simulink model "PMLSM_CDL_MFAC_FFDLc"  (R2023a)
settings: Solver=VariableStepAuto  StartTime=0.0  StopTime=1  RelTol=1e-3
libraries: spsIGBTDiodeLib x6, spsVoltageMeasurementLib x3, slpidlib x2, spsDCVoltageSourceLib x1, simulink x1, spspowerguiLib x1
settings Model: SimulationMode=accelerator  Creator=ComeCross  LastModifiedBy=Administrator
settings SolverCC: ZeroCrossAlgorithm=Adaptive
settings DataIOCC: Refine=10
settings OptimizationCC: ReuseModelBlockBuffer=off
settings DebuggingCC: IgnoredZcDiagnostic=none

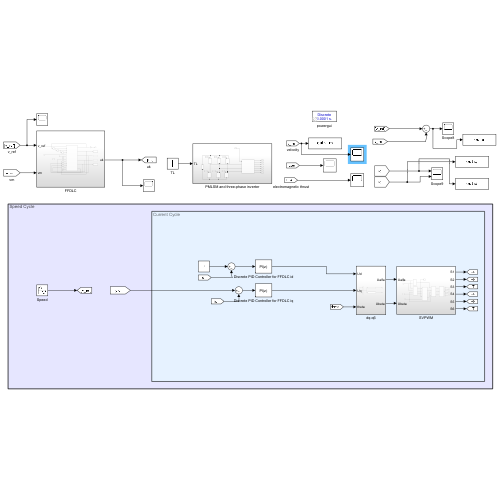
[thumbnail: Simulink's stored preview of the top-level diagram]
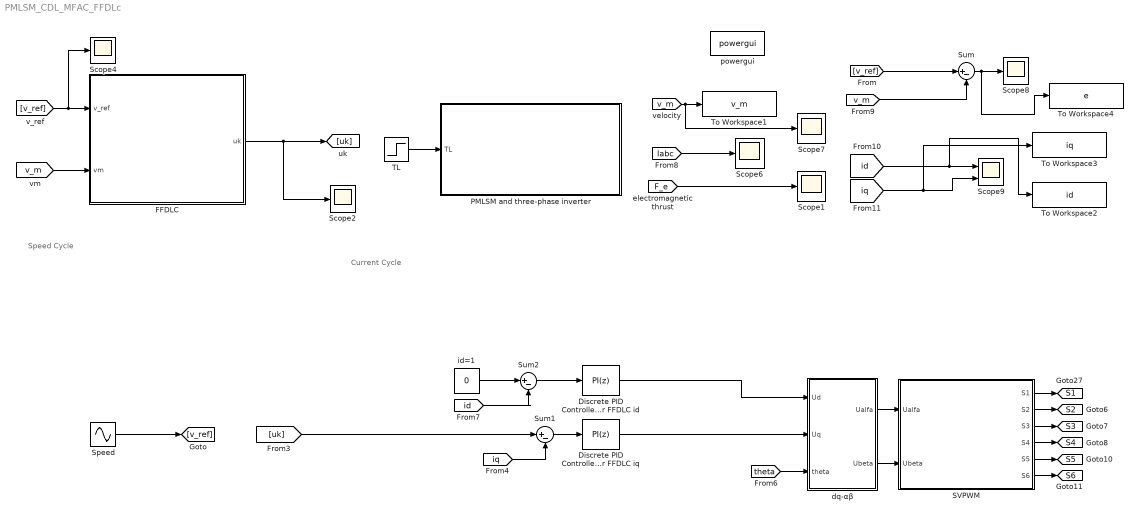
== system PMLSM_CDL_MFAC_FFDLc ==
  note: Speed Cycle
  note: Current Cycle
  Discrete PID Controller for FFDLC id : slpidlib/PID Controller  Controller=PI  Form=Parallel  TimeDomain=Discrete-time  UseExternalTs=off  SampleTime=1e-4  IntegratorMethod=Forward Euler  FilterMethod=Forward Euler  ControllerParametersSource=internal  P=1400  I=2400  UseKiTs=off  D=30  N=100  UseFilter=on  TunerSelectOption=Frequency Response Based  InitialConditionSource=internal  InitialConditionForIntegrator=0  InitialConditionForFilter=0  DifferentiatorICPrevScaledInput=0  ExternalReset=none  TrackingMode=off  Kt=1  LimitOutput=off  SatLimitsSource=internal  UpperSaturationLimit=inf  LowerSaturationLimit=-inf  LinearizeAsGain=off  AntiWindupMode=none  Kb=1  LimitIntegrator=off  UpperIntegratorSaturationLimit=inf  LowerIntegratorSaturationLimit=-inf  POutMin=[]  POutMax=[]  IOutMin=[]  IOutMax=[]  DOutMin=[]  DOutMax=[]  NOutMin=[]  NOutMax=[]  SumOutMin=[]  SumOutMax=[]  SaturationOutMin=[]  SaturationOutMax=[]  PParamMin=[]  PParamMax=[]  IParamMin=[]  IParamMax=[]  DParamMin=[]  DParamMax=[]  NParamMin=[]  NParamMax=[]  KbParamMin=[]  KbParamMax=[]  KtParamMin=[]  KtParamMax=[]  KbOutMin=[]  KbOutMax=[]  KtOutMin=[]  KtOutMax=[]  IntegratorOutMin=[]  IntegratorOutMax=[]  FilterOutMin=[]  FilterOutMax=[]  SumI1OutMin=[]  SumI1OutMax=[]  SumI2OutMin=[]  SumI2OutMax=[]  SumI3OutMin=[]  SumI3OutMax=[]  SumI4OutMin=[]  SumI4OutMax=[]  SumDOutMin=[]  SumDOutMax=[]  DifferentiatorOutMin=[]  DifferentiatorOutMax=[]  FilterDiffOutCoefMin=[]  FilterDiffOutCoefMax=[]  ReciprocalOutMin=[]  ReciprocalOutMax=[]  SumDenOutMin=[]  SumDenOutMax=[]  SumNumOutMin=[]  SumNumOutMax=[]  DivideOutMin=[]  DivideOutMax=[]  UdiffTsProdOutMin=[]  UdiffTsProdOutMax=[]  NTsProdOutMin=[]  NTsProdOutMax=[]  UintegralTsProdOutMin=[]  UintegralTsProdOutMax=[]  UngainTsProdOutMin=[]  UngainTsProdOutMax=[]  ClampingZeroOutDataTypeStr=Inherit: Inherit via back propagation  ClampingZeroOutMin=[]  ClampingZeroOutMax=[]  FilterDenConstantOutDataTypeStr=Inherit: Inherit via back propagation  FilterDenConstantOutMin=[]  FilterDenConstantOutMax=[]  PCopyOutDataTypeStr=Inherit: Inherit via back propagation  PCopyOutMin=[]  PCopyOutMax=[]  NCopyOutDataTypeStr=Inherit: Inherit via back propagation  NCopyOutMin=[]  NCopyOutMax=[]  IntegratorContinuousStateAttributes=''  IntegratorStateMustResolveToSignalObject=off  IntegratorRTWStateStorageClass=Auto  FilterContinuousStateAttributes=''  FilterStateMustResolveToSignalObject=off  FilterRTWStateStorageClass=Auto  ParallelPVariant=InternalParameters  IdealPVariant=Disabled  IVariant=InternalParameters  DVariant=Disabled  IntegratorVariant=Discrete  SatVariant=Disabled  AWVariant=Passthrough  PCopyVariant=Disabled  TRVariant=Disabled  FdbkBlocksVariant=Forward  IdealPFdbkVariant=Disabled  SatFdbkVariant=Disabled  DerivativeFilterVariant=Disabled  NVariant=Disabled  NCopyVariant=Disabled_SignalSpec  FilterICVariant=Disabled  IntegratorICVariant=InternalICs  ExternalResetVariant=Disabled  TRSumVariant=Passthrough  SumFdbkVariant=Disabled  SumVariant=Sum_PI  TsampFilterVariant=InternalTs  TsampNgainVariant=Passthrough  TsampIntegralVariant=Disabled_SignalSpec  ExternalSaturationOutDataTypeStr=Inherit: Same as second input
      settings: LibrarySourceBlock=simulink/Discrete/Discrete PID Controller
  Discrete PID Controller for FFDLC iq : slpidlib/PID Controller  Controller=PI  Form=Parallel  TimeDomain=Discrete-time  UseExternalTs=off  SampleTime=1e-4  IntegratorMethod=Forward Euler  FilterMethod=Forward Euler  ControllerParametersSource=internal  P=1400  I=2400  UseKiTs=off  D=30  N=100  UseFilter=on  TunerSelectOption=Frequency Response Based  InitialConditionSource=internal  InitialConditionForIntegrator=0  InitialConditionForFilter=0  DifferentiatorICPrevScaledInput=0  ExternalReset=none  TrackingMode=off  Kt=1  LimitOutput=off  SatLimitsSource=internal  UpperSaturationLimit=inf  LowerSaturationLimit=-inf  LinearizeAsGain=off  AntiWindupMode=none  Kb=1  LimitIntegrator=off  UpperIntegratorSaturationLimit=inf  LowerIntegratorSaturationLimit=-inf  POutMin=[]  POutMax=[]  IOutMin=[]  IOutMax=[]  DOutMin=[]  DOutMax=[]  NOutMin=[]  NOutMax=[]  SumOutMin=[]  SumOutMax=[]  SaturationOutMin=[]  SaturationOutMax=[]  PParamMin=[]  PParamMax=[]  IParamMin=[]  IParamMax=[]  DParamMin=[]  DParamMax=[]  NParamMin=[]  NParamMax=[]  KbParamMin=[]  KbParamMax=[]  KtParamMin=[]  KtParamMax=[]  KbOutMin=[]  KbOutMax=[]  KtOutMin=[]  KtOutMax=[]  IntegratorOutMin=[]  IntegratorOutMax=[]  FilterOutMin=[]  FilterOutMax=[]  SumI1OutMin=[]  SumI1OutMax=[]  SumI2OutMin=[]  SumI2OutMax=[]  SumI3OutMin=[]  SumI3OutMax=[]  SumI4OutMin=[]  SumI4OutMax=[]  SumDOutMin=[]  SumDOutMax=[]  DifferentiatorOutMin=[]  DifferentiatorOutMax=[]  FilterDiffOutCoefMin=[]  FilterDiffOutCoefMax=[]  ReciprocalOutMin=[]  ReciprocalOutMax=[]  SumDenOutMin=[]  SumDenOutMax=[]  SumNumOutMin=[]  SumNumOutMax=[]  DivideOutMin=[]  DivideOutMax=[]  UdiffTsProdOutMin=[]  UdiffTsProdOutMax=[]  NTsProdOutMin=[]  NTsProdOutMax=[]  UintegralTsProdOutMin=[]  UintegralTsProdOutMax=[]  UngainTsProdOutMin=[]  UngainTsProdOutMax=[]  ClampingZeroOutDataTypeStr=Inherit: Inherit via back propagation  ClampingZeroOutMin=[]  ClampingZeroOutMax=[]  FilterDenConstantOutDataTypeStr=Inherit: Inherit via back propagation  FilterDenConstantOutMin=[]  FilterDenConstantOutMax=[]  PCopyOutDataTypeStr=Inherit: Inherit via back propagation  PCopyOutMin=[]  PCopyOutMax=[]  NCopyOutDataTypeStr=Inherit: Inherit via back propagation  NCopyOutMin=[]  NCopyOutMax=[]  IntegratorContinuousStateAttributes=''  IntegratorStateMustResolveToSignalObject=off  IntegratorRTWStateStorageClass=Auto  FilterContinuousStateAttributes=''  FilterStateMustResolveToSignalObject=off  FilterRTWStateStorageClass=Auto  ParallelPVariant=InternalParameters  IdealPVariant=Disabled  IVariant=InternalParameters  DVariant=Disabled  IntegratorVariant=Discrete  SatVariant=Disabled  AWVariant=Passthrough  PCopyVariant=Disabled  TRVariant=Disabled  FdbkBlocksVariant=Forward  IdealPFdbkVariant=Disabled  SatFdbkVariant=Disabled  DerivativeFilterVariant=Disabled  NVariant=Disabled  NCopyVariant=Disabled_SignalSpec  FilterICVariant=Disabled  IntegratorICVariant=InternalICs  ExternalResetVariant=Disabled  TRSumVariant=Passthrough  SumFdbkVariant=Disabled  SumVariant=Sum_PI  TsampFilterVariant=InternalTs  TsampNgainVariant=Passthrough  TsampIntegralVariant=Disabled_SignalSpec  ExternalSaturationOutDataTypeStr=Inherit: Same as second input
      settings: LibrarySourceBlock=simulink/Discrete/Discrete PID Controller
  FFDLC : Subsystem
  PMLSM and three-phase inverter : Subsystem
  SVPWM : Subsystem
  Scope{1..2,4,6..8} (6 alike) : Scope
  Scope9 : Scope  NumInputPorts=2
  Speed : Sin  Amplitude=2  Frequency=10  SampleTime=0
  Sum : Sum  Inputs=|+-
  Sum1 : Sum  Inputs=|+-
  Sum2 : Sum  Inputs=|+-
  TL : Step  Time=0.2  SampleTime=1e-4
  To Workspace1 : ToWorkspace  VariableName=v_m  SaveFormat=Timeseries  SampleTime=-1
  To Workspace2 : ToWorkspace  VariableName=id  SaveFormat=Structure With Time  SampleTime=-1
  To Workspace3 : ToWorkspace  VariableName=iq  SaveFormat=Structure With Time  SampleTime=-1
  To Workspace4 : ToWorkspace  VariableName=e  SaveFormat=Structure With Time  SampleTime=-1
  dq-αβ : Subsystem
  id=1 : Constant  Value=0
  powergui : spspowerguiLib/powergui  Priority=1  SimulationMode=Discrete  SampleTime=1e-4  frequency=60  Iterations=50  frequencyindice=0  Pbase=100e6  ErrMax=1e-4  UnitsV=kV  UnitsW=MW  buscounter=0  FunctionMessages=off  echomessages=off  EnableUseOfTLC=off  CurrentSourceSwitches=off  DisableSnubberDevices=off  DisableRonSwitches=off  DisableVfSwitches=off  DisplayEquations=off  AutomaticDiscreteSolvers=off  SolverType=Tustin  Interpol=off  ExternalGateDelay=off  methode=off  Ts=0  x0status=blocks  SPID=off  SwTol=0  HookPort=off  NonlinearTolerance=1e-4  nMaxIteration=100  ContinueOnMaxIteration=off  RestoreLinks=warning  ResistiveCurrentMeasurement=off  Frange=[0:2:500]  Ylog=off  Xlog=on  ShowGrid=off  save=off  variable=ZData  structure=0  ZoomFFT=off  StartTime=0.0  cycles=1  DisplayStyle=1  fundamental=60  FreqAxis=off  MaxFrequency=1000  frequencyindicesteady=1  RmsSteady=1  display=off
  tag scope: S1=global, S2=global, S3=global, S4=global, S5=global, S6=global
  wires:
  [v_m] -> Scope7/1, To Workspace1/1
  [Iabc] -> Scope6/1
  [F_e] -> Scope1/1
  SVPWM/6(S6) -> [S6]
  [theta] -> dq-αβ/3(theta)
  SVPWM/5(S5) -> [S5]
  SVPWM/3(S3) -> [S3]
  SVPWM/1(S1) -> [S1]
  dq-αβ/2(Ubeta) -> SVPWM/2(Ubeta)
  SVPWM/4(S4) -> [S4]
  dq-αβ/1(Ualfa) -> SVPWM/1(Ualfa)
  SVPWM/2(S2) -> [S2]
  TL/1 -> PMLSM and three-phase inverter/1(TL)
  Speed/1 -> [v_ref]
  [v_ref] -> Scope4/1, FFDLC/1(v_ref)
  [v_m] -> FFDLC/2(vm)
  FFDLC/1(uk) -> [uk], Scope2/1
  [iq] -> Sum1/2
  Discrete PID Controller for FFDLC id/1 -> dq-αβ/1(Ud)
  id=1/1 -> Sum2/1
  [id] -> Sum2/2
  [v_ref] -> Sum/1
  [v_m] -> Sum/2
  Sum/1 -> To Workspace4/1, Scope8/1
  [id] -> To Workspace2/1, Scope9/1
  [iq] -> To Workspace3/1, Scope9/2
  Sum1/1 -> Discrete PID Controller for FFDLC iq/1
  Sum2/1 -> Discrete PID Controller for FFDLC id/1
  [uk] -> Sum1/1
  Discrete PID Controller for FFDLC iq/1 -> dq-αβ/2(Uq)

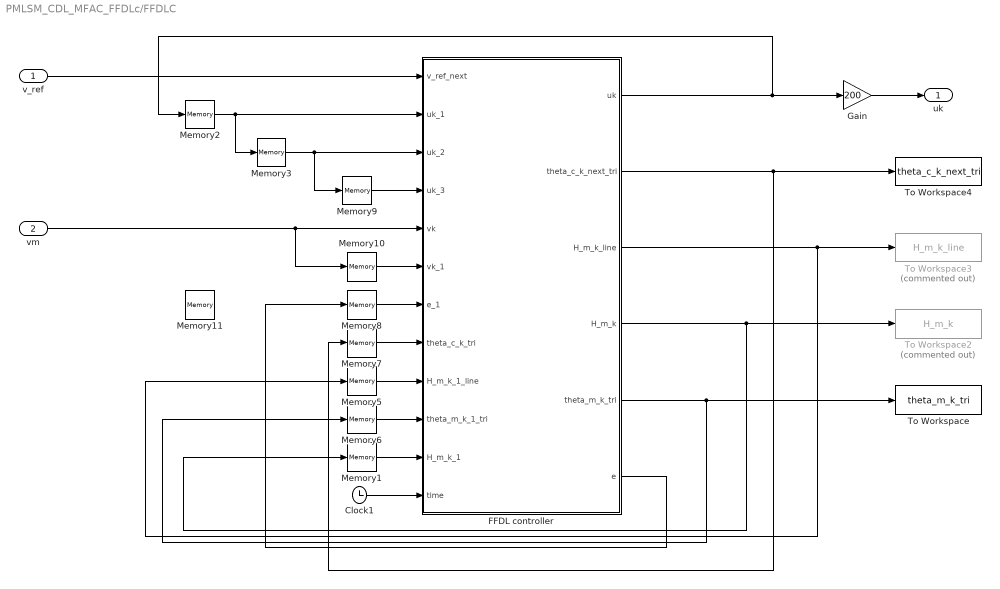
== system PMLSM_CDL_MFAC_FFDLc/FFDLC ==
  v_ref : Inport
  vm : Inport  Port=2
  Clock1 : Clock
  FFDL controller : MATLAB Function  TreatAsAtomicUnit=on
  Gain : Gain  Gain=200
  Memory1 : Memory  InitialCondition=[0.001,0.001,0]'  InheritSampleTime=on
  Memory10 : Memory  InitialCondition=[0]  InheritSampleTime=on
  Memory11 : Memory  InitialCondition=[0.0000]  InheritSampleTime=on
  Memory2 : Memory  InitialCondition=[0.0001]  InheritSampleTime=on
  Memory3 : Memory  InitialCondition=[0.0000]  InheritSampleTime=on
  Memory5 : Memory  InitialCondition=[0.0001,0.000]'  InheritSampleTime=on
  Memory6 : Memory  InitialCondition=[0.006,0.000,-0.000]'  InheritSampleTime=on  LinearizeAsDelay=on
  Memory7 : Memory  InitialCondition=[-0.0048,0.0001,0]'  InheritSampleTime=on
  Memory8 : Memory  InitialCondition=[0.000]  InheritSampleTime=on
  Memory9 : Memory  InitialCondition=[0.00]  InheritSampleTime=on
  To Workspace : ToWorkspace  VariableName=theta_m_k_tri  SaveFormat=Structure With Time  SampleTime=1e-4
      settings: MaxDataPoints=150000
  To Workspace2 : ToWorkspace  Commented=on  VariableName=H_m_k  SaveFormat=Structure With Time  SampleTime=1e-4
  To Workspace3 : ToWorkspace  Commented=on  VariableName=H_m_k_line  SaveFormat=Structure With Time  SampleTime=1e-4
  To Workspace4 : ToWorkspace  VariableName=theta_c_k_next_tri  SaveFormat=Structure With Time  SampleTime=1e-4
      settings: MaxDataPoints=150000
  uk : Outport
  wires:
  FFDL controller/2(theta_c_k_next_tri) -> Memory7/1, To Workspace4/1
  Memory3/1 -> Memory9/1, FFDL controller/3(uk_2)
  vm/1 -> Memory10/1, FFDL controller/5(vk)
  FFDL controller/1(uk) -> Memory2/1, Gain/1
  Memory2/1 -> FFDL controller/2(uk_1), Memory3/1
  FFDL controller/3(H_m_k_line) -> Memory5/1, To Workspace3/1
  FFDL controller/4(H_m_k) -> Memory1/1, To Workspace2/1
  FFDL controller/5(theta_m_k_tri) -> Memory6/1, To Workspace/1
  Memory9/1 -> FFDL controller/4(uk_3)
  v_ref/1 -> FFDL controller/1(v_ref_next)
  Memory10/1 -> FFDL controller/6(vk_1)
  FFDL controller/6(e) -> Memory8/1
  Memory8/1 -> FFDL controller/7(e_1)
  Memory7/1 -> FFDL controller/8(theta_c_k_tri)
  Memory5/1 -> FFDL controller/9(H_m_k_1_line)
  Memory6/1 -> FFDL controller/10(theta_m_k_1_tri)
  Memory1/1 -> FFDL controller/11(H_m_k_1)
  Gain/1 -> uk/1
  Clock1/1 -> FFDL controller/12(time)

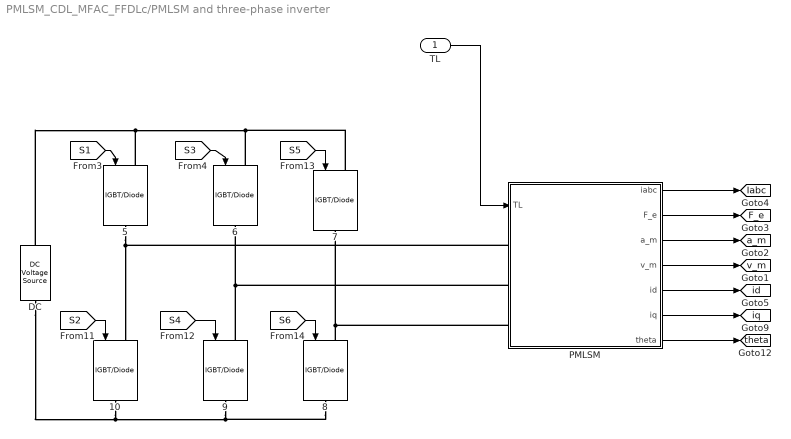
== system PMLSM_CDL_MFAC_FFDLc/PMLSM and three-phase inverter ==
  TL : Inport
  {5..10} (6 alike) : spsIGBTDiodeLib/IGBT//Diode  Ron=1e-3  Rs=5000  Cs=inf  Measurements=off
  DC : spsDCVoltageSourceLib/DC Voltage Source  Amplitude=220*(2^0.5)  Measurements=None
  PMLSM : Subsystem  mask{Rs=2.6, Ld=0.0267, Lq=0.0267, Ff=0.24, pi=3.1416, Pn=2, M=6.6, Bv=0.2, tao=0.018}
      mask prompts: Rs "resistance(Rs):"; Ld "d-axis inductance(Ld):"; Lq "d-axis inductance(Lq):"; Ff "flux linkage(Ff):"; Pn "number of pole pairs(Pn):"; M "mass(M):"; Bv "Viscosity(Bv):"; tao "pole distance(tao):"
  tag scope: F_e=global, Iabc=global, a_m=global, id=global, iq=global, theta=global, v_m=global
  wires:
  PMLSM/5(id) -> [id]
  [S6] -> 8/1
  PMLSM/6(iq) -> [iq]
  PMLSM/7(theta) -> [theta]
  PMLSM/2(F_e) -> [F_e]
  [S2] -> 10/1
  PMLSM/3(a_m) -> [a_m]
  [S5] -> 7/1
  [S1] -> 5/1
  PMLSM/4(v_m) -> [v_m]
  PMLSM/1(iabc) -> [Iabc]
  [S4] -> 9/1
  [S3] -> 6/1
  TL/1 -> PMLSM/1(TL)
  connections:
  PMLSM/LConn2 -- 9/LConn1 -- 6/RConn1
  PMLSM/LConn1 -- 5/RConn1 -- 10/LConn1
  10/RConn1 -- DC/LConn1 -- 8/RConn1 -- 9/RConn1
  8/LConn1 -- PMLSM/LConn3 -- 7/RConn1
  DC/RConn1 -- 5/LConn1 -- 6/LConn1 -- 7/LConn1

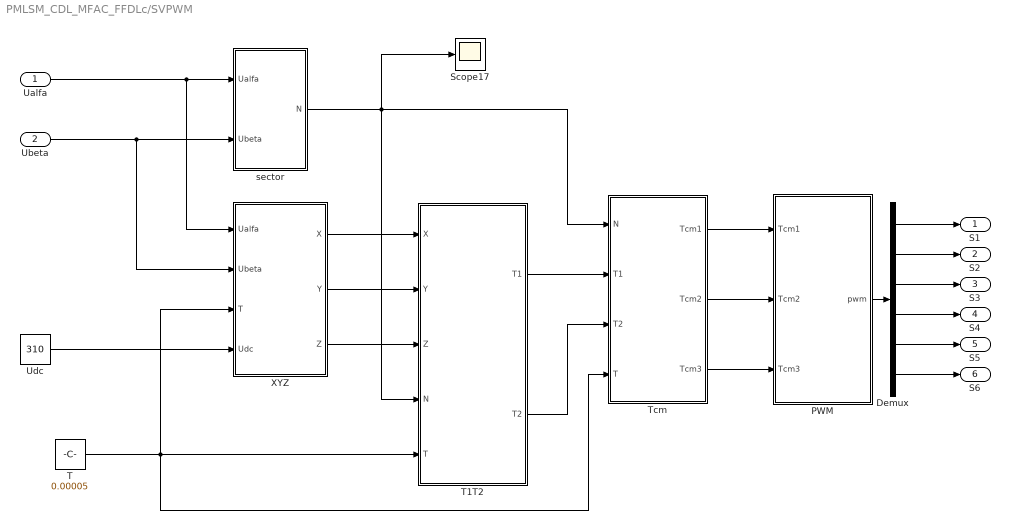
== system PMLSM_CDL_MFAC_FFDLc/SVPWM ==
  Ualfa : Inport
  Ubeta : Inport  Port=2
  Demux : Demux  Outputs=6
  PWM : Subsystem
  Scope17 : Scope
  T : Constant  Value=0.00005
  T1T2 : Subsystem
  Tcm : Subsystem
  Udc : Constant  Value=310
  XYZ : Subsystem
  sector : Subsystem
  S1 : Outport  VectorParamsAs1DForOutWhenUnconnected=off
  S2 : Outport  Port=2  VectorParamsAs1DForOutWhenUnconnected=off
  S3 : Outport  Port=3  VectorParamsAs1DForOutWhenUnconnected=off
  S4 : Outport  Port=4  VectorParamsAs1DForOutWhenUnconnected=off
  S5 : Outport  Port=5  VectorParamsAs1DForOutWhenUnconnected=off
  S6 : Outport  Port=6  VectorParamsAs1DForOutWhenUnconnected=off
  wires:
  Ualfa/1 -> XYZ/1(Ualfa), sector/1(Ualfa)
  Ubeta/1 -> sector/2(Ubeta), XYZ/2(Ubeta)
  Udc/1 -> XYZ/4(Udc)
  XYZ/1(X) -> T1T2/1(X)
  XYZ/2(Y) -> T1T2/2(Y)
  XYZ/3(Z) -> T1T2/3(Z)
  T/1 -> T1T2/5(T), Tcm/4(T), XYZ/3(T)
  sector/1(N) -> Scope17/1, Tcm/1(N), T1T2/4(N)
  T1T2/1(T1) -> Tcm/2(T1)
  T1T2/2(T2) -> Tcm/3(T2)
  Tcm/1(Tcm1) -> PWM/1(Tcm1)
  Tcm/2(Tcm2) -> PWM/2(Tcm2)
  Tcm/3(Tcm3) -> PWM/3(Tcm3)
  PWM/1(pwm) -> Demux/1
  Demux/1 -> S1/1
  Demux/2 -> S2/1
  Demux/3 -> S3/1
  Demux/4 -> S4/1
  Demux/5 -> S5/1
  Demux/6 -> S6/1

== system PMLSM_CDL_MFAC_FFDLc/dq-αβ ==
  Ud : Inport
  Uq : Inport  Port=2
  theta : Inport  Port=3
  Fcn1 : Fcn  Expr=u(1)*cos(u(3))-u(2)*sin(u(3))
  Fcn2 : Fcn  Expr=u(1)*sin(u(3))+u(2)*cos(u(3))
  Mux1 : Mux  Inputs=3
  Ualfa : Outport  VectorParamsAs1DForOutWhenUnconnected=off
  Ubeta : Outport  Port=2  VectorParamsAs1DForOutWhenUnconnected=off
  wires:
  Mux1/1 -> Fcn2/1, Fcn1/1
  Ud/1 -> Mux1/1
  Uq/1 -> Mux1/2
  theta/1 -> Mux1/3
  Fcn1/1 -> Ualfa/1
  Fcn2/1 -> Ubeta/1

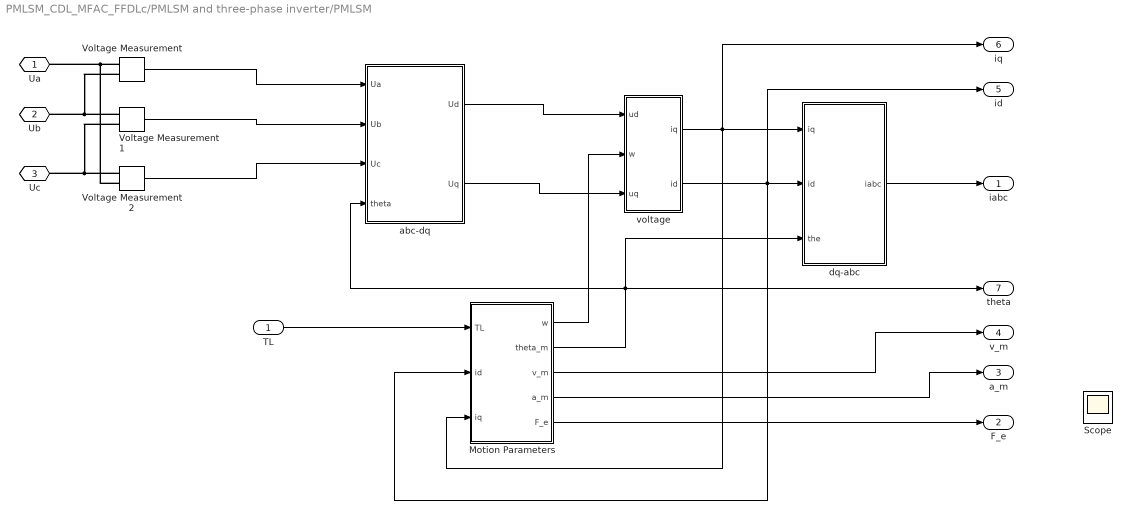
== system PMLSM_CDL_MFAC_FFDLc/PMLSM and three-phase inverter/PMLSM ==
  TL : Inport
  Motion Parameters : Subsystem
  Scope : Scope
  Voltage Measurement : spsVoltageMeasurementLib/Voltage Measurement  PhasorSimulation=off  OutputType=Complex  PSBequivalent=0
  Voltage Measurement1 : spsVoltageMeasurementLib/Voltage Measurement  PhasorSimulation=off  OutputType=Complex  PSBequivalent=0
  Voltage Measurement2 : spsVoltageMeasurementLib/Voltage Measurement  PhasorSimulation=off  OutputType=Complex  PSBequivalent=0
  abc-dq : Subsystem
  dq-abc : Subsystem
  voltage : Subsystem
  Ua : PMIOPort  Side=Left
  Ub : PMIOPort  Port=2  Side=Left
  Uc : PMIOPort  Port=3  Side=Left
  iabc : Outport  VectorParamsAs1DForOutWhenUnconnected=off
  F_e : Outport  Port=2  VectorParamsAs1DForOutWhenUnconnected=off
  a_m : Outport  Port=3  VectorParamsAs1DForOutWhenUnconnected=off
  v_m : Outport  Port=4  VectorParamsAs1DForOutWhenUnconnected=off
  id : Outport  Port=5  VectorParamsAs1DForOutWhenUnconnected=off
  iq : Outport  Port=6  VectorParamsAs1DForOutWhenUnconnected=off
  theta : Outport  Port=7  VectorParamsAs1DForOutWhenUnconnected=off
  wires:
  Voltage Measurement/1 -> abc-dq/1(Ua)
  Voltage Measurement1/1 -> abc-dq/2(Ub)
  Voltage Measurement2/1 -> abc-dq/3(Uc)
  voltage/1(iq) -> iq/1, Motion Parameters/3(iq), dq-abc/1(iq)
  voltage/2(id) -> id/1, Motion Parameters/2(id), dq-abc/2(id)
  TL/1 -> Motion Parameters/1(TL)
  Motion Parameters/1(w) -> voltage/2(w)
  Motion Parameters/2(theta_m) -> abc-dq/4(theta), dq-abc/3(the), theta/1
  dq-abc/1(iabc) -> iabc/1
  Motion Parameters/3(v_m) -> v_m/1
  Motion Parameters/4(a_m) -> a_m/1
  Motion Parameters/5(F_e) -> F_e/1
  abc-dq/1(Ud) -> voltage/1(ud)
  abc-dq/2(Uq) -> voltage/3(uq)
  connections:
  Voltage Measurement/LConn1 -- Voltage Measurement2/LConn2 -- Ua/RConn1
  Voltage Measurement/LConn2 -- Voltage Measurement1/LConn1 -- Ub/RConn1
  Voltage Measurement1/LConn2 -- Uc/RConn1 -- Voltage Measurement2/LConn1

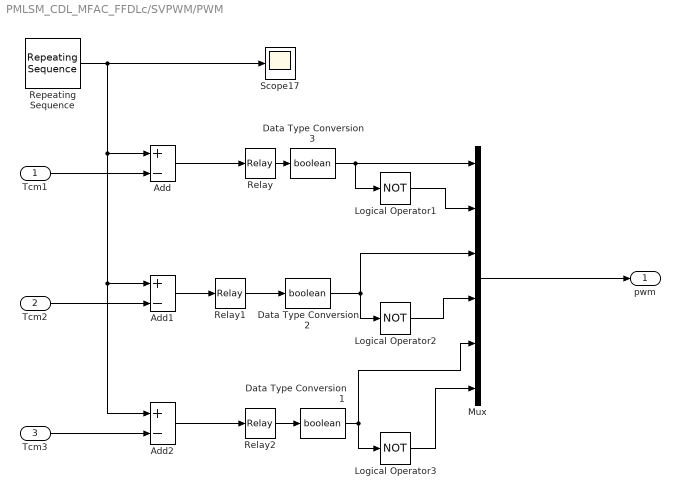
== system PMLSM_CDL_MFAC_FFDLc/SVPWM/PWM ==
  Tcm1 : Inport
  Tcm2 : Inport  Port=2
  Tcm3 : Inport  Port=3
  Add : Sum  Inputs=+-
  Add1 : Sum  Inputs=+-
  Add2 : Sum  Inputs=+-
  Data Type Conversion1 : DataTypeConversion  OutDataTypeStr=boolean  SaturateOnIntegerOverflow=off  RndMeth=Floor
  Data Type Conversion2 : DataTypeConversion  OutDataTypeStr=boolean  SaturateOnIntegerOverflow=off  RndMeth=Floor
  Data Type Conversion3 : DataTypeConversion  OutDataTypeStr=boolean  SaturateOnIntegerOverflow=off  RndMeth=Floor
  Logical Operator1 : Logic  Operator=NOT  AllPortsSameDT=off  OutDataTypeStr=boolean
  Logical Operator2 : Logic  Operator=NOT  AllPortsSameDT=off  OutDataTypeStr=boolean
  Logical Operator3 : Logic  Operator=NOT  AllPortsSameDT=off  OutDataTypeStr=boolean
  Mux : Mux  Inputs=6
  Relay : Relay  OnSwitchValue=2e-10  OffSwitchValue=-2e-10
  Relay1 : Relay  OnSwitchValue=2e-10  OffSwitchValue=-2e-10
  Relay2 : Relay  OnSwitchValue=2e-10  OffSwitchValue=-2e-10
  Repeating Sequence : simulink/Sources/Repeating Sequence  rep_seq_t=[0 0.000025 0.00005]  rep_seq_y=[0 0.000025 0]
  Scope17 : Scope
  pwm : Outport  VectorParamsAs1DForOutWhenUnconnected=off
  wires:
  Tcm1/1 -> Add/2
  Tcm2/1 -> Add1/2
  Tcm3/1 -> Add2/2
  Repeating Sequence/1 -> Scope17/1, Add1/1, Add2/1, Add/1
  Add/1 -> Relay/1
  Add1/1 -> Relay1/1
  Add2/1 -> Relay2/1
  Relay/1 -> Data Type Conversion3/1
  Relay2/1 -> Data Type Conversion1/1
  Relay1/1 -> Data Type Conversion2/1
  Logical Operator1/1 -> Mux/2
  Logical Operator2/1 -> Mux/4
  Logical Operator3/1 -> Mux/6
  Mux/1 -> pwm/1
  Data Type Conversion2/1 -> Mux/3, Logical Operator2/1
  Data Type Conversion3/1 -> Mux/1, Logical Operator1/1
  Data Type Conversion1/1 -> Logical Operator3/1, Mux/5

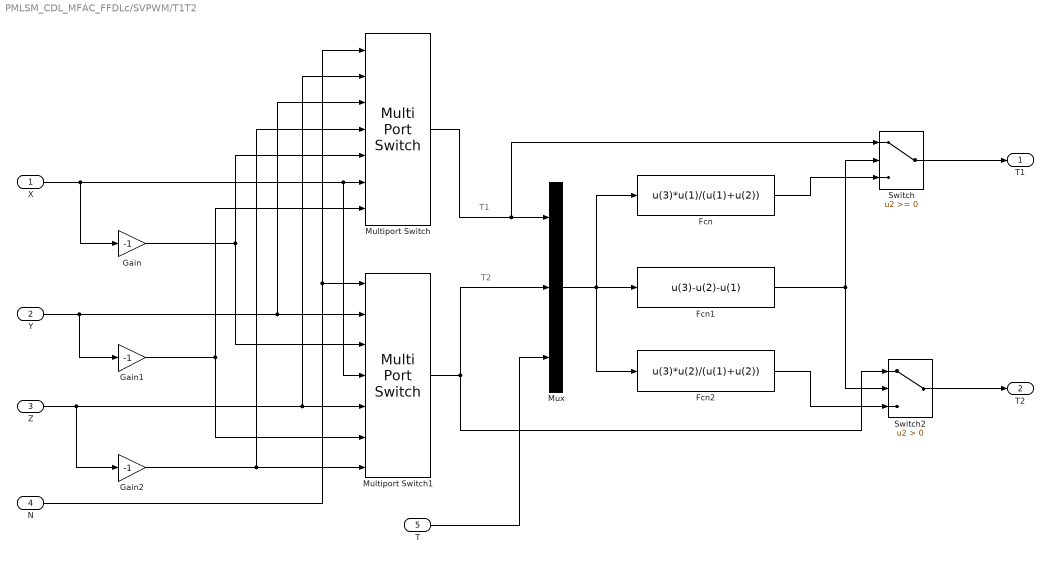
== system PMLSM_CDL_MFAC_FFDLc/SVPWM/T1T2 ==
  note: T2
  note: T1
  X : Inport
  Y : Inport  Port=2
  Z : Inport  Port=3
  N : Inport  Port=4
  T : Inport  Port=5
  Fcn : Fcn  Expr=u(3)*u(1)/(u(1)+u(2))
  Fcn1 : Fcn  Expr=u(3)-u(2)-u(1)
  Fcn2 : Fcn  Expr=u(3)*u(2)/(u(1)+u(2))
  Gain : Gain  Gain=-1
  Gain1 : Gain  Gain=-1
  Gain2 : Gain  Gain=-1
  Multiport Switch : MultiPortSwitch  Inputs=6  DiagnosticForDefault=None  SaturateOnIntegerOverflow=off  InputSameDT=off
  Multiport Switch1 : MultiPortSwitch  Inputs=6  DiagnosticForDefault=None  SaturateOnIntegerOverflow=off  InputSameDT=off
  Mux : Mux  Inputs=3
  Switch : Switch  SaturateOnIntegerOverflow=off  InputSameDT=off
  Switch2 : Switch  Criteria=u2 > Threshold  SaturateOnIntegerOverflow=off  InputSameDT=off
  T1 : Outport  VectorParamsAs1DForOutWhenUnconnected=off
  T2 : Outport  Port=2  VectorParamsAs1DForOutWhenUnconnected=off
  wires:
  N/1 -> Multiport Switch1/1, Multiport Switch/1
  Z/1 -> Gain2/1, Multiport Switch1/5, Multiport Switch/2
  Y/1 -> Multiport Switch1/2, Multiport Switch/3, Gain1/1
  Gain2/1 -> Multiport Switch1/7, Multiport Switch/4
  Gain/1 -> Multiport Switch1/3, Multiport Switch/5
  X/1 -> Gain/1, Multiport Switch/6, Multiport Switch1/4
  Gain1/1 -> Multiport Switch1/6, Multiport Switch/7
  Multiport Switch/1 -> Switch/1, Mux/1
  Multiport Switch1/1 -> Switch2/1, Mux/2
  T/1 -> Mux/3
  Mux/1 -> Fcn/1, Fcn1/1, Fcn2/1
  Fcn1/1 -> Switch2/2, Switch/2
  Fcn/1 -> Switch/3
  Fcn2/1 -> Switch2/3
  Switch/1 -> T1/1
  Switch2/1 -> T2/1

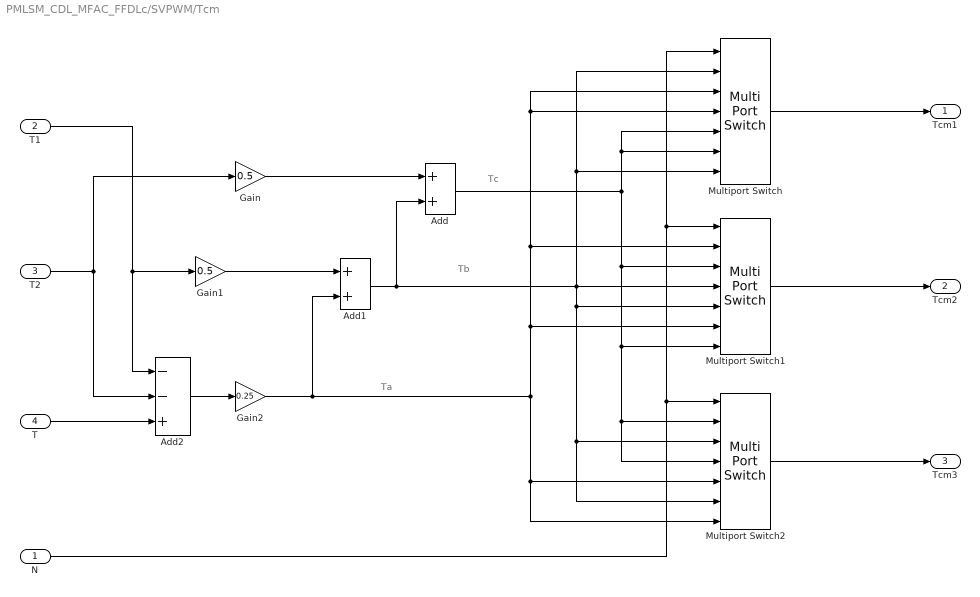
== system PMLSM_CDL_MFAC_FFDLc/SVPWM/Tcm ==
  note: Tc
  note: Tb
  note: Ta
  N : Inport
  T1 : Inport  Port=2
  T2 : Inport  Port=3
  T : Inport  Port=4
  Add : Sum
  Add1 : Sum
  Add2 : Sum  Inputs=--+
  Gain : Gain  Gain=0.5
  Gain1 : Gain  Gain=0.5
  Gain2 : Gain  Gain=0.25
  Multiport Switch : MultiPortSwitch  Inputs=6  DiagnosticForDefault=None  SaturateOnIntegerOverflow=off  InputSameDT=off
  Multiport Switch1 : MultiPortSwitch  Inputs=6  DiagnosticForDefault=None  SaturateOnIntegerOverflow=off  InputSameDT=off
  Multiport Switch2 : MultiPortSwitch  Inputs=6  DiagnosticForDefault=None  SaturateOnIntegerOverflow=off  InputSameDT=off
  Tcm1 : Outport  VectorParamsAs1DForOutWhenUnconnected=off
  Tcm2 : Outport  Port=2  VectorParamsAs1DForOutWhenUnconnected=off
  Tcm3 : Outport  Port=3  VectorParamsAs1DForOutWhenUnconnected=off
  wires:
  T/1 -> Add2/3
  T2/1 -> Gain/1, Add2/2
  T1/1 -> Gain1/1, Add2/1
  Add2/1 -> Gain2/1
  Gain2/1 -> Add1/2, Multiport Switch1/6, Multiport Switch1/2, Multiport Switch/4, Multiport Switch/3, Multiport Switch2/7, Multiport Switch2/5
  Gain1/1 -> Add1/1
  Add1/1 -> Multiport Switch2/6, Multiport Switch2/3, Multiport Switch1/5, Multiport Switch1/4, Multiport Switch/7, Multiport Switch/2, Add/2
  Gain/1 -> Add/1
  N/1 -> Multiport Switch2/1, Multiport Switch/1, Multiport Switch1/1
  Add/1 -> Multiport Switch2/4, Multiport Switch2/2, Multiport Switch1/7, Multiport Switch1/3, Multiport Switch/6, Multiport Switch/5
  Multiport Switch/1 -> Tcm1/1
  Multiport Switch1/1 -> Tcm2/1
  Multiport Switch2/1 -> Tcm3/1

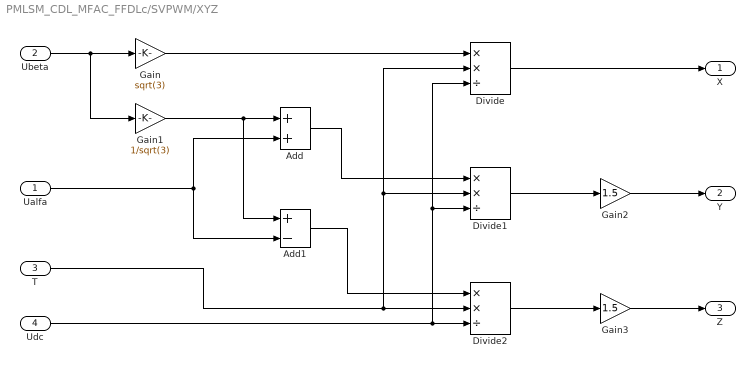
== system PMLSM_CDL_MFAC_FFDLc/SVPWM/XYZ ==
  Ualfa : Inport
  Ubeta : Inport  Port=2
  T : Inport  Port=3
  Udc : Inport  Port=4
  Add : Sum
  Add1 : Sum  Inputs=+-
  Divide : Product  Inputs=**/
  Divide1 : Product  Inputs=**/
  Divide2 : Product  Inputs=**/
  Gain : Gain  Gain=sqrt(3)
  Gain1 : Gain  Gain=1/sqrt(3)
  Gain2 : Gain  Gain=1.5
  Gain3 : Gain  Gain=1.5
  X : Outport  VectorParamsAs1DForOutWhenUnconnected=off
  Y : Outport  Port=2  VectorParamsAs1DForOutWhenUnconnected=off
  Z : Outport  Port=3  VectorParamsAs1DForOutWhenUnconnected=off
  wires:
  Ubeta/1 -> Gain1/1, Gain/1
  Gain/1 -> Divide/1
  Divide/1 -> X/1
  Divide1/1 -> Gain2/1
  Gain2/1 -> Y/1
  Divide2/1 -> Gain3/1
  Gain3/1 -> Z/1
  Udc/1 -> Divide1/3, Divide/3, Divide2/3
  T/1 -> Divide1/2, Divide/2, Divide2/2
  Gain1/1 -> Add1/1, Add/1
  Ualfa/1 -> Add1/2, Add/2
  Add/1 -> Divide1/1
  Add1/1 -> Divide2/1

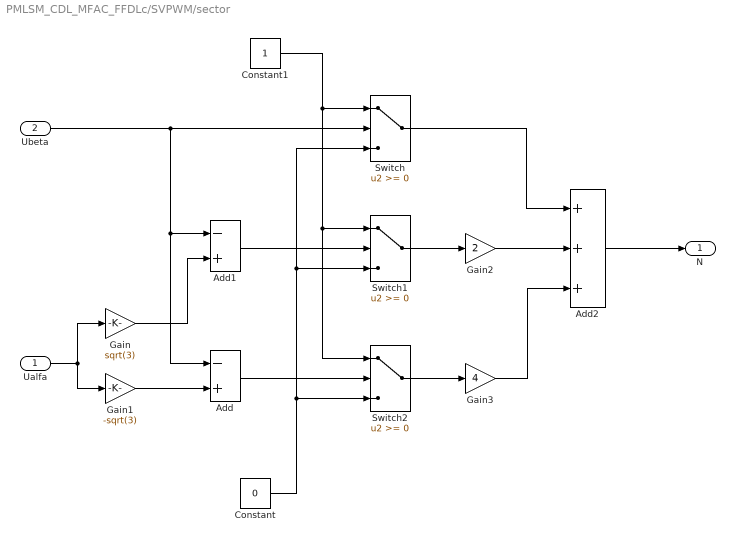
== system PMLSM_CDL_MFAC_FFDLc/SVPWM/sector ==
  Ualfa : Inport
  Ubeta : Inport  Port=2
  Add : Sum  Inputs=-+
  Add1 : Sum  Inputs=-+
  Add2 : Sum  Inputs=+++
  Constant : Constant  Value=0
  Constant1 : Constant
  Gain : Gain  Gain=sqrt(3)
  Gain1 : Gain  Gain=-sqrt(3)
  Gain2 : Gain  Gain=2
  Gain3 : Gain  Gain=4
  Switch : Switch  SaturateOnIntegerOverflow=off  InputSameDT=off
  Switch1 : Switch  SaturateOnIntegerOverflow=off  InputSameDT=off
  Switch2 : Switch  SaturateOnIntegerOverflow=off  InputSameDT=off
  N : Outport  VectorParamsAs1DForOutWhenUnconnected=off
  wires:
  Ubeta/1 -> Add1/1, Add/1, Switch/2
  Constant1/1 -> Switch/1, Switch1/1, Switch2/1
  Constant/1 -> Switch2/3, Switch1/3, Switch/3
  Add/1 -> Switch2/2
  Add1/1 -> Switch1/2
  Switch1/1 -> Gain2/1
  Switch2/1 -> Gain3/1
  Switch/1 -> Add2/1
  Gain2/1 -> Add2/2
  Gain3/1 -> Add2/3
  Add2/1 -> N/1
  Ualfa/1 -> Gain/1, Gain1/1
  Gain1/1 -> Add/2
  Gain/1 -> Add1/2

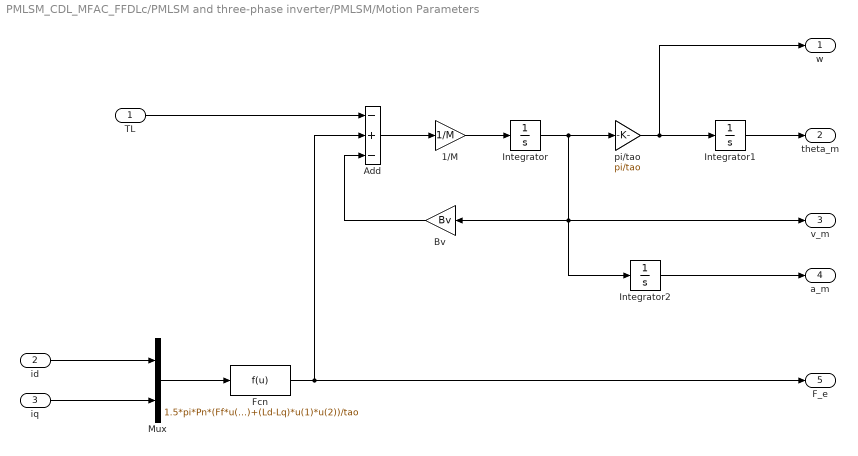
== system PMLSM_CDL_MFAC_FFDLc/PMLSM and three-phase inverter/PMLSM/Motion Parameters ==
  TL : Inport
  id : Inport  Port=2
  iq : Inport  Port=3
  1/M : Gain  Gain=1/M
  Add : Sum  Inputs=-+-
  Bv : Gain  Gain=Bv
  Fcn : Fcn  Expr=1.5*pi*Pn*(Ff*u(2)+(Ld-Lq)*u(1)*u(2))/tao
  Integrator : Integrator
  Integrator1 : Integrator
  Integrator2 : Integrator
  Mux : Mux  Inputs=2
  pi/tao : Gain  Gain=pi/tao
  w : Outport  VectorParamsAs1DForOutWhenUnconnected=off
  theta_m : Outport  Port=2  VectorParamsAs1DForOutWhenUnconnected=off
  v_m : Outport  Port=3  VectorParamsAs1DForOutWhenUnconnected=off
  a_m : Outport  Port=4  VectorParamsAs1DForOutWhenUnconnected=off
  F_e : Outport  Port=5  VectorParamsAs1DForOutWhenUnconnected=off
  wires:
  TL/1 -> Add/1
  Fcn/1 -> F_e/1, Add/2
  Bv/1 -> Add/3
  Add/1 -> 1/M/1
  1/M/1 -> Integrator/1
  Integrator/1 -> Integrator2/1, v_m/1, Bv/1, pi/tao/1
  Integrator2/1 -> a_m/1
  pi/tao/1 -> w/1, Integrator1/1
  Integrator1/1 -> theta_m/1
  id/1 -> Mux/1
  iq/1 -> Mux/2
  Mux/1 -> Fcn/1

== system PMLSM_CDL_MFAC_FFDLc/PMLSM and three-phase inverter/PMLSM/abc-dq ==
  Ua : Inport
  Ub : Inport  Port=2
  Uc : Inport  Port=3
  theta : Inport  Port=4
  Fcn : Fcn  Expr=sqrt(2/3)*(cos(u(4))*u(1)+cos(u(4)-2*pi/3)*u(2)+cos(u(4)+2*pi/3)*u(3))
  Fcn1 : Fcn  Expr=-sqrt(2/3)*(sin(u(4))*u(1)+sin(u(4)-2*pi/3)*u(2)+sin(u(4)+2*pi/3)*u(3))
  Mux : Mux
  Ud : Outport  VectorParamsAs1DForOutWhenUnconnected=off
  Uq : Outport  Port=2  VectorParamsAs1DForOutWhenUnconnected=off
  wires:
  Uc/1 -> Mux/3
  theta/1 -> Mux/4
  Ub/1 -> Mux/2
  Ua/1 -> Mux/1
  Mux/1 -> Fcn1/1, Fcn/1
  Fcn/1 -> Ud/1
  Fcn1/1 -> Uq/1

== system PMLSM_CDL_MFAC_FFDLc/PMLSM and three-phase inverter/PMLSM/dq-abc ==
  iq : Inport
  id : Inport  Port=2
  the : Inport  Port=3
  Fcn : Fcn  Expr=sqrt(2/3)*(cos(u(3))*u(2)-sin(u(3))*u(1))
  Fcn1 : Fcn  Expr=sqrt(2/3)*(cos(u(3)-2*pi/3)*u(2)-sin(u(3)-2*pi/3)*u(1))
  Fcn2 : Fcn  Expr=sqrt(2/3)*(cos(u(3)+2*pi/3)*u(2)-sin(u(3)+2*pi/3)*u(1))
  Mux : Mux  Inputs=3
  Mux1 : Mux  Inputs=3
  iabc : Outport  VectorParamsAs1DForOutWhenUnconnected=off
  wires:
  Mux/1 -> Fcn2/1, Fcn/1, Fcn1/1
  Fcn1/1 -> Mux1/2
  Fcn/1 -> Mux1/1
  Fcn2/1 -> Mux1/3
  Mux1/1 -> iabc/1
  iq/1 -> Mux/1
  id/1 -> Mux/2
  the/1 -> Mux/3

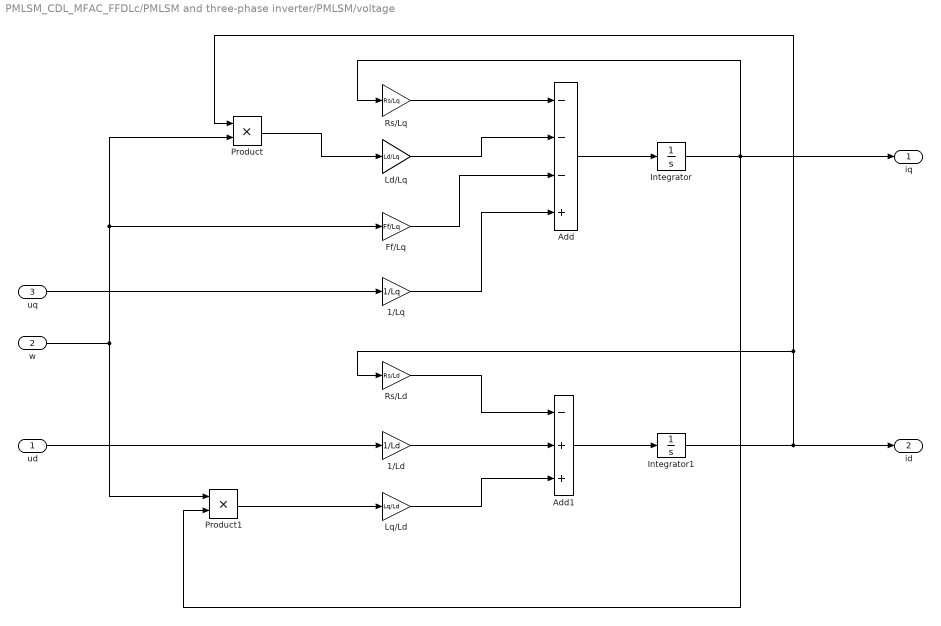
== system PMLSM_CDL_MFAC_FFDLc/PMLSM and three-phase inverter/PMLSM/voltage ==
  ud : Inport
  w : Inport  Port=2
  uq : Inport  Port=3
  1/Ld : Gain  Gain=1/Ld
  1/Lq : Gain  Gain=1/Lq
  Add : Sum  Inputs=---+
  Add1 : Sum  Inputs=-++
  Ff/Lq : Gain  Gain=Ff/Lq
  Integrator : Integrator
  Integrator1 : Integrator
  Ld/Lq : Gain  Gain=Ld/Lq
  Lq/Ld : Gain  Gain=Lq/Ld
  Product : Product
  Product1 : Product
  Rs/Ld : Gain  Gain=Rs/Ld
  Rs/Lq : Gain  Gain=Rs/Lq
  iq : Outport  VectorParamsAs1DForOutWhenUnconnected=off
  id : Outport  Port=2  VectorParamsAs1DForOutWhenUnconnected=off
  wires:
  ud/1 -> 1/Ld/1
  1/Ld/1 -> Add1/2
  w/1 -> Product1/1, Ff/Lq/1, Product/2
  Add/1 -> Integrator/1
  Add1/1 -> Integrator1/1
  Integrator1/1 -> id/1, Product/1, Rs/Ld/1
  Integrator/1 -> Product1/2, iq/1, Rs/Lq/1
  Product1/1 -> Lq/Ld/1
  Lq/Ld/1 -> Add1/3
  Rs/Ld/1 -> Add1/1
  uq/1 -> 1/Lq/1
  1/Lq/1 -> Add/4
  Ff/Lq/1 -> Add/3
  Product/1 -> Ld/Lq/1
  Ld/Lq/1 -> Add/2
  Rs/Lq/1 -> Add/1

== matlab function PMLSM_CDL_MFAC_FFDLc/FFDLC/FFDL controller ==
  data: v_ref_next input; uk_1 input; uk output; uk_2 input; uk_3 input; vk input; vk_1 input; e_1 input; theta_c_k_tri input; H_m_k_1_line input; theta_m_k_1_tri input; H_m_k_1 input; theta_c_k_next_tri output; H_m_k_line output; H_m_k output; theta_m_k_tri output; e output; time input
function [uk,theta_c_k_next_tri,H_m_k_line,H_m_k,theta_m_k_tri,e]  = fcn(v_ref_next,uk_1,uk_2,uk_3,vk,vk_1,e_1,theta_c_k_tri,H_m_k_1_line,theta_m_k_1_tri,H_m_k_1,time)
Lu=2;
Ly=1;
Lc=1;
Le=2;
eita_m=0.5;
eita_c=0.5;
%60000
lamda_m=60000;  %penalty of changing rate
%0.1
lamda_c=0.1;
sample_time=1e-4;
bu=0.01;
bm=0.009;
%0.009
bc=0.08;
%0.006


%k=round(time/sample_time);
%disp(k);
% uk0=0.001;
% vk0=0.001;
% theta_c_k_next_tri0=[-0.004,0.001,0]';
% H_m_k_line0=[0.001,0.0001]';
% theta_m_k_tri0=[-0.003,0.001,0.001]';


% if k<=1
%     delta_u_1=uk_1-uk_2;
%     %delta_u_2=uk_2-uk_3;
%     e=v_ref_next-vk;
%     delta_e=e-e_1;
%     H_c_k_line=[(-1*e),delta_e,delta_u_1]';
%     uk = uk_1 + theta_c_k_tri'*H_c_k_line;
% 
%     %vk=vk0;
%     theta_c_k_next_tri=theta_c_k_next_tri0;
% 
%     H_m_k_line=H_m_k_line0;
% 
%     H_m_k_line=[uk_1,vk]';
% 
%     H_m_k=[uk,H_m_k_line']';
% 
%     theta_m_k_tri=theta_m_k_tri0;
%     
%     uk=uk0;
% %     k=k_next+1;
% else
    
    delta_u_1=uk_1-uk_2;
    delta_u_2=uk_2-uk_3;
    e=v_ref_next-vk;
    delta_e=e-e_1;
    H_c_k_line=[(-1*e),delta_e,delta_u_1]';

    H_m_k_line=[uk_1,vk]';

    delta_H_m_k_line=H_m_k_line-H_m_k_1_line;

    uk = uk_1 + theta_c_k_tri'*H_c_k_line;

    H_m_k=[uk,H_m_k_line']';

    delta_H_m_k_1=H_m_k-H_m_k_1;

    if uk>bu
        uk=bu;
    end
    if uk<-bu
        uk=-bu;
    end

    theta_m_k_tri=theta_m_k_1_tri + eita_m*((vk-vk_1)/(lamda_m+power(norm(delta_H_m_k_1),2)))*delta_H_m_k_1 - eita_m*((theta_m_k_1_tri'*delta_H_m_k_1)/(lamda_m+power(norm(delta_H_m_k_1),2)))*delta_H_m_k_1;
    if norm(theta_m_k_tri) >= bm
        theta_m_k_tri=theta_m_k_1_tri;
        %disp("1");
    end
    
    theta_c_k_next_tri=(1-eita_c)*theta_c_k_tri + eita_c*((theta_m_k_tri(1,1)*(v_ref_next-vk-theta_m_k_tri(2:3,1)'*delta_H_m_k_line)*H_c_k_line)/((lamda_c+power(theta_m_k_tri(1),2))*power(norm(H_c_k_line),2)));

    if norm(H_c_k_line)==0 || norm(theta_c_k_next_tri)>bc
        theta_c_k_next_tri=theta_m_k_tri;
        %disp('2');
    end
end
